simulink model "ATV7_SIMULINK"  (R2021a)
settings: Solver=VariableStepAuto  StartTime=0.0  StopTime=1.5  RelTol=1e-3
settings Model: Creator=Home  LastModifiedBy=Home

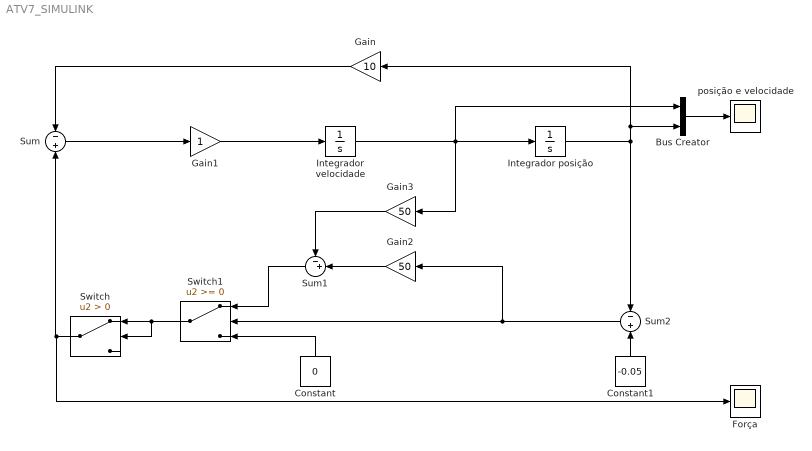
== system ATV7_SIMULINK ==
  Bus Creator : BusCreator  Inputs=2
  Constant : Constant  Value=0
  Constant1 : Constant  Value=-0.05
  Força : Scope
  Gain : Gain  Gain=10
  Gain1 : Gain
  Gain2 : Gain  Gain=50
  Gain3 : Gain  Gain=50
  Integrador posição : Integrator  InitialCondition=0.05
  Integrador velocidade : Integrator  InitialCondition=-0.5
  Sum : Sum  Inputs=-|+
  Sum1 : Sum  Inputs=-+|
  Sum2 : Sum  Inputs=-|+
  Switch : Switch  Criteria=u2 > Threshold
  Switch1 : Switch
  posição e velocidade : Scope
  wires:
  Gain1/1 -> Integrador velocidade/1
  Integrador velocidade/1 -> Gain3/1, Bus Creator/1, Integrador posição/1
  Gain/1 -> Sum/1
  Integrador posição/1 -> Bus Creator/2, Gain/1, Sum2/1
  Sum/1 -> Gain1/1
  Bus Creator/1 -> posição e velocidade/1
  Gain3/1 -> Sum1/1
  Gain2/1 -> Sum1/2
  Sum1/1 -> Switch1/1
  Switch1/1 -> Switch/2, Switch/1
  Switch/1 -> Força/1, Sum/2
  Sum2/1 -> Gain2/1, Switch1/2
  Constant1/1 -> Sum2/2
  Constant/1 -> Switch1/3
